simulink model "model4"  (R2022b)
settings: Solver=FixedStepAuto  StartTime=0.0  StopTime=10  FixedStep=0.00001  RelTol=1e-3
values from neighbouring files (symbols this model uses):
  a21 = 1/2/m * x30^2 * FemP1/FemP2^2 * exp(-x10/FemP2)    [init.m]    (also in proj.m)
  a23 = -1/m * x30 * FemP1/FemP2 * exp(-x10/FemP2)    [init.m]    (also in proj.m)
  a31 = 1/f1 * exp(x10/f2) * (ki*u10 + ci - x30)    [init.m]    (also in proj.m)
  a33 = -f2/f1 * exp(x10/f2)    [init.m]    (also in proj.m)
  b31 = ki * f2/f1 * exp(x10/f2)    [init.m]    (also in proj.m)
  g = 9.81    [init.m]    (also in proj.m)
  K = place(A, B(:, 1), [-28, -60, -90])    [init.m]    (also in proj.m)
  xd = d-bd    [init.m]    (also in proj.m)
settings Model: Creator=TheZl  LastModifiedBy=minekuba

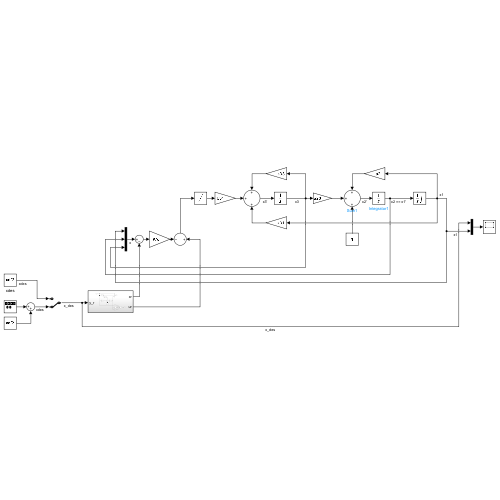
[thumbnail: Simulink's stored preview of the top-level diagram]
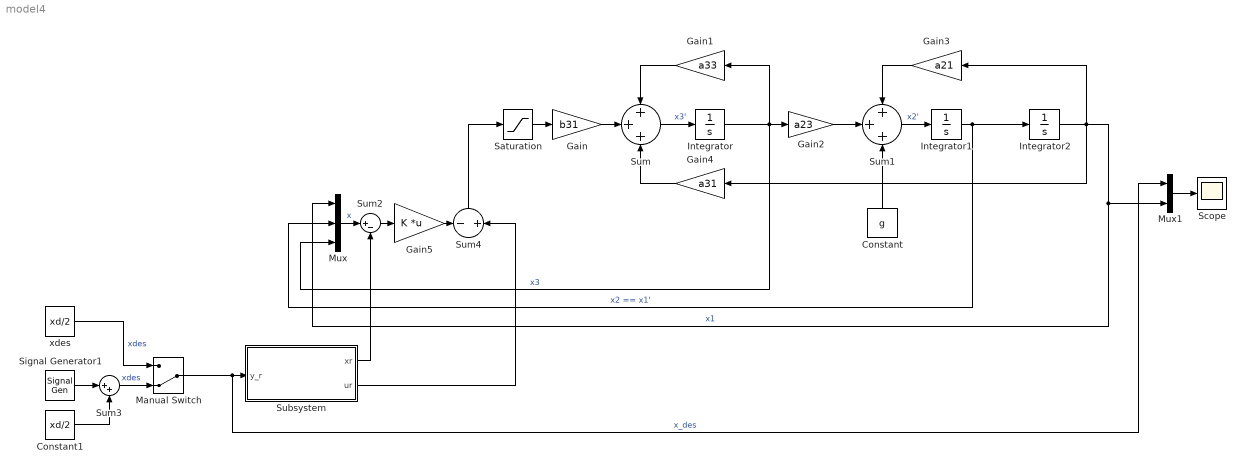
== system model4 ==
  Constant : Constant  Value=g
  Constant1 : Constant  Value=xd/2
  Gain : Gain  Gain=b31
  Gain1 : Gain  Gain=a33
  Gain2 : Gain  Gain=a23
  Gain3 : Gain  Gain=a21
  Gain4 : Gain  Gain=a31
  Gain5 : Gain  Gain=K  Multiplication=Matrix(K*u)
  Integrator : Integrator
  Integrator1 : Integrator
  Integrator2 : Integrator  InitialCondition=xd  LimitOutput=on  UpperSaturationLimit=xd  LowerSaturationLimit=0
  Manual Switch : ManualSwitch  CurrentSetting=0
  Mux : Mux  Inputs=3
  Mux1 : Mux  Inputs=2
  Saturation : Saturate  UpperLimit=1  LowerLimit=0
  Scope : Scope
  Signal Generator1 : SignalGenerator  Amplitude=xd/12  Frequency=0.1
  Subsystem : Subsystem
  Sum : Sum  Inputs=+++
  Sum1 : Sum  Inputs=+++
  Sum2 : Sum  Inputs=|+-
  Sum3 : Sum  Inputs=|++
  Sum4 : Sum  Inputs=-|+
  xdes : Constant  Value=xd/2
  wires:
  Subsystem/2(ur) -> Sum4/2
  Gain5/1 -> Sum4/1
  Sum4/1 -> Saturation/1
  Integrator/1 -> Mux/3, Gain1/1, Gain2/1  "x3"
  Saturation/1 -> Gain/1
  Constant/1 -> Sum1/3
  Gain4/1 -> Sum/3
  Integrator1/1 -> Mux/2, Integrator2/1  "x2 == x1'"
  Sum/1 -> Integrator/1  "x3'"
  Gain1/1 -> Sum/1
  Gain3/1 -> Sum1/1
  Integrator2/1 -> Mux/1, Mux1/2, Gain4/1, Gain3/1  "x1"
  Sum1/1 -> Integrator1/1  "x2'"
  Gain/1 -> Sum/2
  Gain2/1 -> Sum1/2
  Manual Switch/1 -> Mux1/1, Subsystem/1(y_r)  "x_des"
  Mux/1 -> Sum2/1  "x"
  Sum2/1 -> Gain5/1
  Subsystem/1(xr) -> Sum2/2
  Mux1/1 -> Scope/1
  Signal Generator1/1 -> Sum3/1
  xdes/1 -> Manual Switch/1  "xdes"
  Constant1/1 -> Sum3/2
  Sum3/1 -> Manual Switch/2  "xdes"

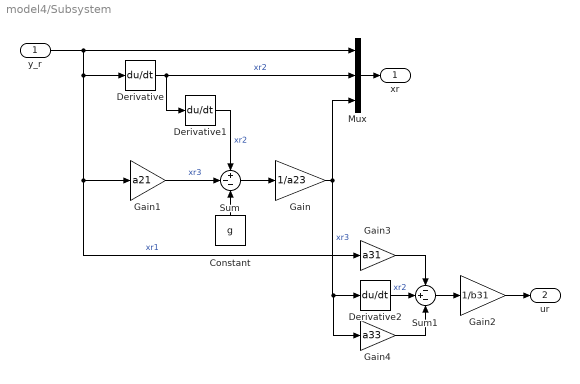
== system model4/Subsystem ==
  y_r : Inport
  Constant : Constant  Value=g
  Derivative : Derivative
  Derivative1 : Derivative
  Derivative2 : Derivative
  Gain : Gain  Gain=1/a23
  Gain1 : Gain  Gain=a21
  Gain2 : Gain  Gain=1/b31
  Gain3 : Gain  Gain=a31
  Gain4 : Gain  Gain=a33
  Mux : Mux  Inputs=3
  Sum : Sum  Inputs=+--
  Sum1 : Sum  Inputs=-+-
  xr : Outport
  ur : Outport  Port=2
  wires:
  Mux/1 -> xr/1
  y_r/1 -> Gain3/1, Gain1/1, Derivative/1, Mux/1  "xr1"
  Derivative/1 -> Derivative1/1, Mux/2  "xr2"
  Gain/1 -> Gain4/1, Derivative2/1, Mux/3  "xr3"
  Derivative1/1 -> Sum/1  "xr2"
  Sum/1 -> Gain/1
  Constant/1 -> Sum/3
  Gain1/1 -> Sum/2  "xr3"
  Gain2/1 -> ur/1
  Sum1/1 -> Gain2/1
  Derivative2/1 -> Sum1/2  "xr2"
  Gain3/1 -> Sum1/1
  Gain4/1 -> Sum1/3
